simulink model "roboterrestreESC"  (R2015b)
settings: Solver=ode1  StartTime=0.0  StopTime=Tsimu  FixedStep=passo  RelTol=1e-3
values from neighbouring files (symbols this model uses):
  h = (v/Rr)/5    (= 0.314159265359)    [initroboterrestreESC.m]
  N = 10    [initroboterrestreESC.m]
  Rr = 2    [initroboterrestreESC.m]
  v = 1*pi*Rr/2    (= 3.14159265359)    [initroboterrestreESC.m]
  x0 = zeros(1,5)'    [initroboterrestreESC.m]
settings Model: Creator=alessandropeixoto  LastModifiedBy=alessandropeixoto

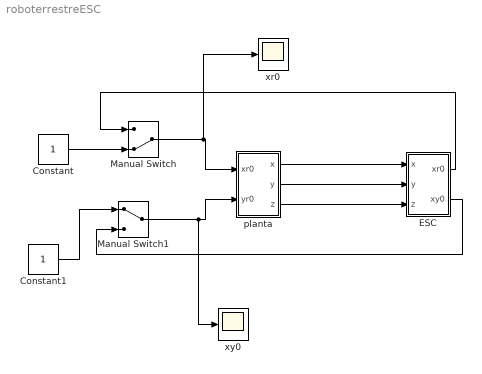
== system roboterrestreESC ==
  Constant : Constant
  Constant1 : Constant
  ESC : Subsystem
  Manual Switch : ManualSwitch  CurrentSetting=0
  Manual Switch1 : ManualSwitch
  planta : Subsystem
  xr0 : Scope
  xy0 : Scope
  wires:
  planta/1(x) -> ESC/1(x)
  planta/2(y) -> ESC/2(y)
  planta/3(z) -> ESC/3(z)
  Manual Switch/1 -> xr0/1, planta/1(xr0)
  Constant/1 -> Manual Switch/2
  ESC/1(xr0) -> Manual Switch/1
  Constant1/1 -> Manual Switch1/1
  ESC/2(xy0) -> Manual Switch1/2
  Manual Switch1/1 -> xy0/1, planta/2(yr0)

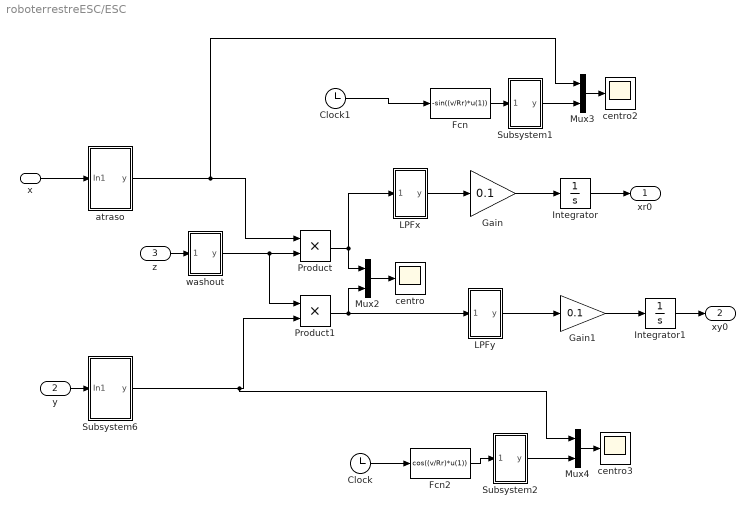
== system roboterrestreESC/ESC ==
  x : Inport
  y : Inport  Port=2
  z : Inport  Port=3
  Clock : Clock
  Clock1 : Clock
  Fcn : Fcn  Expr=-sin((v/Rr)*u(1))
  Fcn2 : Fcn  Expr=cos((v/Rr)*u(1))
  Gain : Gain  Gain=0.1
  Gain1 : Gain  Gain=0.1
  Integrator : Integrator  InitialCondition=1
  Integrator1 : Integrator  InitialCondition=1
  LPFx : Subsystem
  LPFy : Subsystem
  Mux2 : Mux  Inputs=2
  Mux3 : Mux  Inputs=2
  Mux4 : Mux  Inputs=2
  Product : Product
  Product1 : Product
  Subsystem1 : Subsystem
  Subsystem2 : Subsystem
  Subsystem6 : Subsystem
  atraso : Subsystem
  centro : Scope
  centro2 : Scope
  centro3 : Scope
  washout : Subsystem
  xr0 : Outport
  xy0 : Outport  Port=2
  wires:
  Subsystem6/1(y) -> Mux4/1, Product1/2
  Gain/1 -> Integrator/1
  LPFy/1(y) -> Gain1/1
  x/1 -> atraso/1(In1)
  z/1 -> washout/1(In1)
  y/1 -> Subsystem6/1(In1)
  Mux4/1 -> centro3/1
  Integrator1/1 -> xy0/1
  Integrator/1 -> xr0/1
  atraso/1(y) -> Mux3/1, Product/1
  Product1/1 -> Mux2/2, LPFy/1(In1)
  Subsystem1/1(y) -> Mux3/2
  Subsystem2/1(y) -> Mux4/2
  Gain1/1 -> Integrator1/1
  Mux3/1 -> centro2/1
  Fcn/1 -> Subsystem1/1(In1)
  Fcn2/1 -> Subsystem2/1(In1)
  Clock/1 -> Fcn2/1
  Clock1/1 -> Fcn/1
  washout/1(y) -> Product1/1, Product/2
  Mux2/1 -> centro/1
  Product/1 -> Mux2/1, LPFx/1(In1)
  LPFx/1(y) -> Gain/1

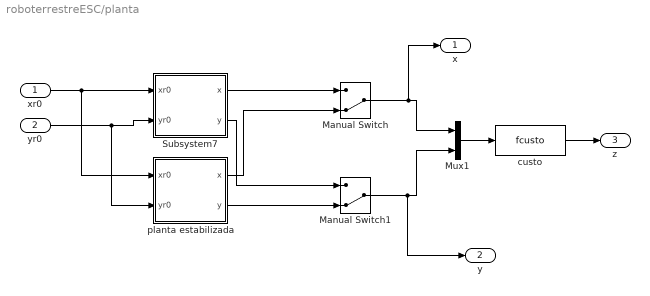
== system roboterrestreESC/planta ==
  xr0 : Inport
  yr0 : Inport  Port=2
  Manual Switch : ManualSwitch  CurrentSetting=0
  Manual Switch1 : ManualSwitch  CurrentSetting=0
  Mux1 : Mux  Inputs=2
  Subsystem7 : Subsystem
  custo : MATLABFcn  MATLABFcn=fcusto
  planta estabilizada : Subsystem
  x : Outport
  y : Outport  Port=2
  z : Outport  Port=3
  wires:
  Manual Switch1/1 -> y/1, Mux1/2
  xr0/1 -> planta estabilizada/1(xr0), Subsystem7/1(xr0)
  yr0/1 -> planta estabilizada/2(yr0), Subsystem7/2("yr0 ")
  planta estabilizada/1(x) -> Manual Switch/2
  custo/1 -> z/1
  Manual Switch/1 -> x/1, Mux1/1
  planta estabilizada/2(y) -> Manual Switch1/2
  Subsystem7/2(y) -> Manual Switch1/1
  Mux1/1 -> custo/1
  Subsystem7/1(x) -> Manual Switch/1

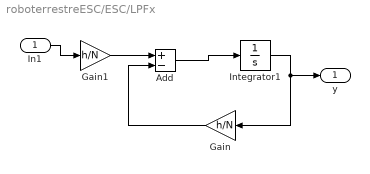
== system roboterrestreESC/ESC/LPFx ==
  In1 : Inport
  Add : Sum  Inputs=+-
  Gain : Gain  Gain=h/N
  Gain1 : Gain  Gain=h/N
  Integrator1 : Integrator
  y : Outport
  wires:
  Add/1 -> Integrator1/1
  In1/1 -> Gain1/1
  Gain/1 -> Add/2
  Integrator1/1 -> y/1, Gain/1
  Gain1/1 -> Add/1

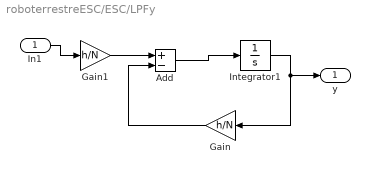
== system roboterrestreESC/ESC/LPFy ==
  In1 : Inport
  Add : Sum  Inputs=+-
  Gain : Gain  Gain=h/N
  Gain1 : Gain  Gain=h/N
  Integrator1 : Integrator
  y : Outport
  wires:
  Add/1 -> Integrator1/1
  In1/1 -> Gain1/1
  Gain/1 -> Add/2
  Integrator1/1 -> y/1, Gain/1
  Gain1/1 -> Add/1

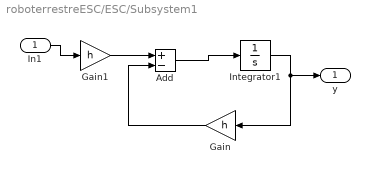
== system roboterrestreESC/ESC/Subsystem1 ==
  In1 : Inport
  Add : Sum  Inputs=+-
  Gain : Gain  Gain=h
  Gain1 : Gain  Gain=h
  Integrator1 : Integrator
  y : Outport
  wires:
  Add/1 -> Integrator1/1
  In1/1 -> Gain1/1
  Gain/1 -> Add/2
  Integrator1/1 -> y/1, Gain/1
  Gain1/1 -> Add/1

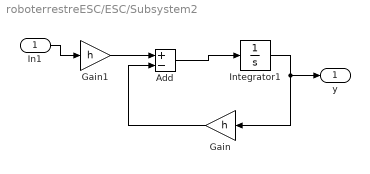
== system roboterrestreESC/ESC/Subsystem2 ==
  In1 : Inport
  Add : Sum  Inputs=+-
  Gain : Gain  Gain=h
  Gain1 : Gain  Gain=h
  Integrator1 : Integrator
  y : Outport
  wires:
  Add/1 -> Integrator1/1
  In1/1 -> Gain1/1
  Gain/1 -> Add/2
  Integrator1/1 -> y/1, Gain/1
  Gain1/1 -> Add/1

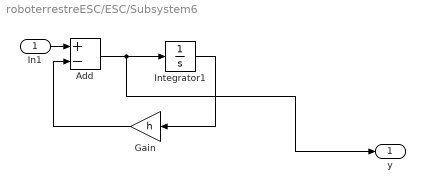
== system roboterrestreESC/ESC/Subsystem6 ==
  In1 : Inport
  Add : Sum  Inputs=+-
  Gain : Gain  Gain=h
  Integrator1 : Integrator
  y : Outport
  wires:
  Add/1 -> y/1, Integrator1/1
  Integrator1/1 -> Gain/1
  In1/1 -> Add/1
  Gain/1 -> Add/2

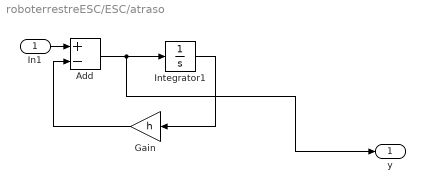
== system roboterrestreESC/ESC/atraso ==
  In1 : Inport
  Add : Sum  Inputs=+-
  Gain : Gain  Gain=h
  Integrator1 : Integrator
  y : Outport
  wires:
  Add/1 -> y/1, Integrator1/1
  Integrator1/1 -> Gain/1
  In1/1 -> Add/1
  Gain/1 -> Add/2

== system roboterrestreESC/ESC/washout ==
  In1 : Inport
  Add : Sum  Inputs=+-
  Gain : Gain  Gain=h
  Integrator1 : Integrator
  y : Outport
  wires:
  Add/1 -> y/1, Integrator1/1
  Integrator1/1 -> Gain/1
  In1/1 -> Add/1
  Gain/1 -> Add/2

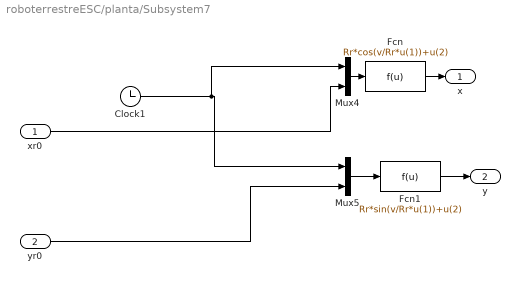
== system roboterrestreESC/planta/Subsystem7 ==
  xr0 : Inport
  "yr0 " : Inport  Port=2
  Clock1 : Clock
  Fcn : Fcn  Expr=Rr*cos(v/Rr*u(1))+u(2)
  Fcn1 : Fcn  Expr=Rr*sin(v/Rr*u(1))+u(2)
  Mux4 : Mux  Inputs=2
  Mux5 : Mux  Inputs=2
  x : Outport
  y : Outport  Port=2
  wires:
  xr0/1 -> Mux4/2
  Mux5/1 -> Fcn1/1
  Fcn1/1 -> y/1
  Mux4/1 -> Fcn/1
  Clock1/1 -> Mux5/1, Mux4/1
  "yr0 "/1 -> Mux5/2
  Fcn/1 -> x/1

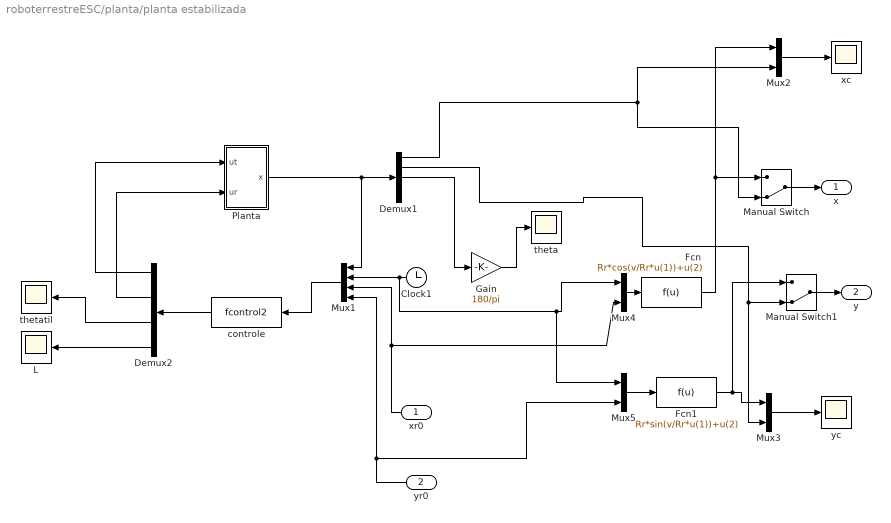
== system roboterrestreESC/planta/planta estabilizada ==
  xr0 : Inport
  yr0 : Inport  Port=2
  Clock1 : Clock
  Demux1 : Demux  Outputs=5
  Demux2 : Demux
  Fcn : Fcn  Expr=Rr*cos(v/Rr*u(1))+u(2)
  Fcn1 : Fcn  Expr=Rr*sin(v/Rr*u(1))+u(2)
  Gain : Gain  Gain=180/pi
  L : Scope
  Manual Switch : ManualSwitch  CurrentSetting=0
  Manual Switch1 : ManualSwitch  CurrentSetting=0
  Mux1 : Mux
  Mux{2..5} (4 alike) : Mux  Inputs=2
  Planta : Subsystem
  controle : MATLABFcn  MATLABFcn=fcontrol2
  theta : Scope
  thetatil : Scope
  xc : Scope
  yc : Scope
  x : Outport
  y : Outport  Port=2
  wires:
  Demux1/1 -> Manual Switch/2, Mux2/2
  controle/1 -> Demux2/1
  Planta/1(x) -> Demux1/1, Mux1/1
  Clock1/1 -> Mux5/1, Mux4/1, Mux1/2
  Demux1/3 -> Gain/1
  Demux2/2 -> Planta/2(ur)
  yr0/1 -> Mux5/2, Mux1/4
  Gain/1 -> theta/1
  Demux2/4 -> L/1
  Mux1/1 -> controle/1
  Demux2/3 -> thetatil/1
  Demux2/1 -> Planta/1(ut)
  xr0/1 -> Mux1/3, Mux4/2
  Mux2/1 -> xc/1
  Fcn/1 -> Manual Switch/1, Mux2/1
  Mux3/1 -> yc/1
  Fcn1/1 -> Manual Switch1/1, Mux3/1
  Mux4/1 -> Fcn/1
  Mux5/1 -> Fcn1/1
  Demux1/2 -> Mux3/2, Manual Switch1/2
  Manual Switch/1 -> x/1
  Manual Switch1/1 -> y/1

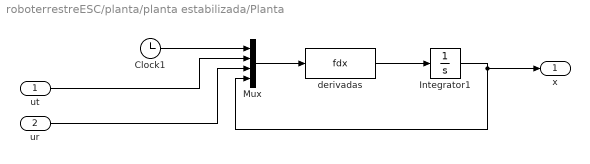
== system roboterrestreESC/planta/planta estabilizada/Planta ==
  ut : Inport
  ur : Inport  Port=2
  Clock1 : Clock
  Integrator1 : Integrator  InitialCondition=x0
  Mux : Mux
  derivadas : MATLABFcn  MATLABFcn=fdx
  x : Outport
  wires:
  ur/1 -> Mux/3
  ut/1 -> Mux/2
  Clock1/1 -> Mux/1
  Mux/1 -> derivadas/1
  Integrator1/1 -> x/1, Mux/4
  derivadas/1 -> Integrator1/1
